simulink model "Efficiency_Map_SR_Validation_Sim"  (R2017b)
settings: Solver=VariableStepAuto  StartTime=0.0  StopTime=10.0  RelTol=1e-3
values from neighbouring files (symbols this model uses):
  ap00 = -69.58    [Efficiency_Map_Validation.m]    (also in Efficiency_Maps.m)
  ap01 = 11.22    [Efficiency_Map_Validation.m]    (also in Efficiency_Maps.m)
  ap02 = -0.1665    [Efficiency_Map_Validation.m]    (also in Efficiency_Maps.m)
  ap03 = 0.0006218    [Efficiency_Map_Validation.m]    (also in Efficiency_Maps.m)
  ap10 = 0.5123    [Efficiency_Map_Validation.m]    (also in Efficiency_Maps.m)
  ap11 = 0.009736    [Efficiency_Map_Validation.m]    (also in Efficiency_Maps.m)
  ap12 = 0.0003316    [Efficiency_Map_Validation.m]    (also in Efficiency_Maps.m)
  ap20 = -0.0007943    [Efficiency_Map_Validation.m]    (also in Efficiency_Maps.m)
  ap21 = -4.587e-07    [Efficiency_Map_Validation.m]    (also in Efficiency_Maps.m)
  ap30 = 3.794e-07    [Efficiency_Map_Validation.m]    (also in Efficiency_Maps.m)
  motor_speed = mtr_speed_rad(j)    [Efficiency_Map_Validation.m]
  motor_torque = mtr_torque(i)    [Efficiency_Map_Validation.m]
settings Model: Creator=Robert Wygant  LastModifiedBy=Robert Wygant

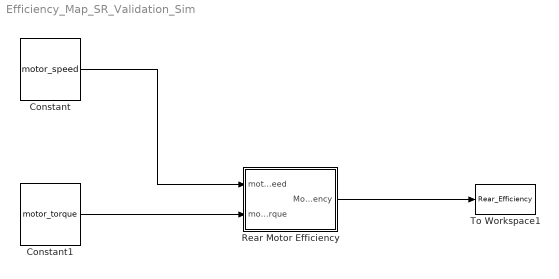
== system Efficiency_Map_SR_Validation_Sim ==
  Constant : Constant  Value=motor_speed
  Constant1 : Constant  Value=motor_torque
  Rear Motor Efficiency : Subsystem
      mask Display:
      | color('green')
      | disp("Motor Efficiency")
  To Workspace1 : ToWorkspace  VariableName=Rear_Efficiency  SampleTime=-1
      settings: MaxDataPoints=1  Save2DSignal=2-D array (concatenate along first dimension)
  wires:
  Constant/1 -> Rear Motor Efficiency/1(motor_speed)
  Constant1/1 -> Rear Motor Efficiency/2(motor_torque)
  Rear Motor Efficiency/1(Motor_efficiency) -> To Workspace1/1

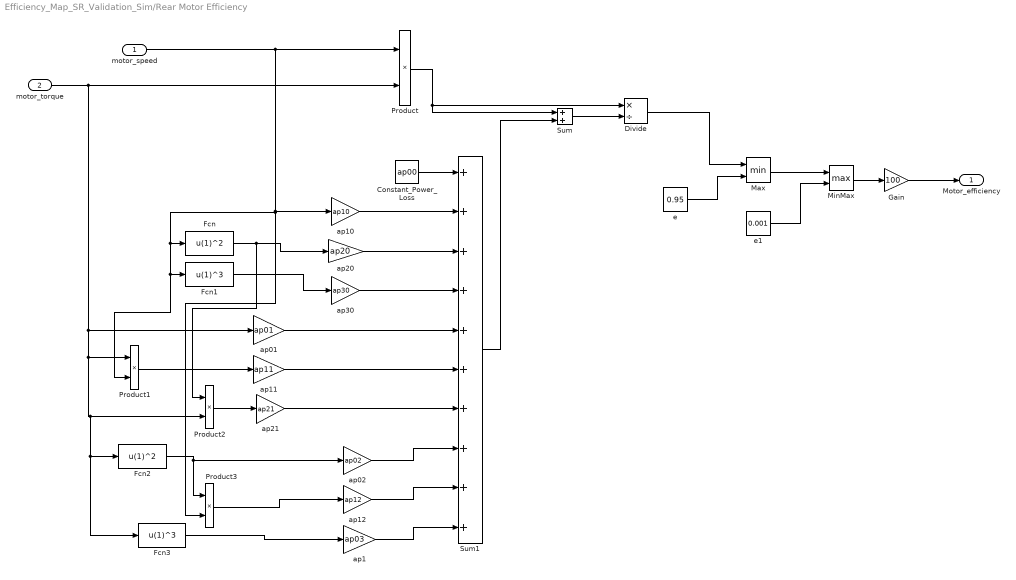
== system Efficiency_Map_SR_Validation_Sim/Rear Motor Efficiency ==
  motor_speed : Inport
  motor_torque : Inport  Port=2
  Constant_Power_Loss : Constant  Value=ap00
  Divide : Product  Inputs=*/
  Fcn : Fcn  Expr=u(1)^2
  Fcn1 : Fcn  Expr=u(1)^3
  Fcn2 : Fcn  Expr=u(1)^2
  Fcn3 : Fcn  Expr=u(1)^3
  Gain : Gain  Gain=100
  Max : MinMax  Inputs=2
  MinMax : MinMax  Function=max  Inputs=2
  Product{,1..3} (4 alike) : Product
  Sum : Sum
  Sum1 : Sum  Inputs=++++++++++
  ap01 : Gain  Gain=ap01
  ap02 : Gain  Gain=ap02
  ap1 : Gain  Gain=ap03
  ap10 : Gain  Gain=ap10
  ap11 : Gain  Gain=ap11
  ap12 : Gain  Gain=ap12
  ap20 : Gain  Gain=ap20
  ap21 : Gain  Gain=ap21
  ap30 : Gain  Gain=ap30
  e : Constant  Value=0.95
  e1 : Constant  Value=0.001
  Motor_efficiency : Outport
  wires:
  e/1 -> Max/2
  Fcn3/1 -> ap1/1
  ap1/1 -> Sum1/10
  ap12/1 -> Sum1/9
  Product3/1 -> ap12/1
  motor_torque/1 -> Product/2, Product1/1, Product2/2, Fcn2/1, Fcn3/1, ap01/1
  ap01/1 -> Sum1/5
  ap11/1 -> Sum1/6
  ap21/1 -> Sum1/7
  ap02/1 -> Sum1/8
  Fcn2/1 -> ap02/1, Product3/1
  Product2/1 -> ap21/1
  Product1/1 -> ap11/1
  ap30/1 -> Sum1/4
  Fcn1/1 -> ap30/1
  Fcn/1 -> ap20/1, Product2/1
  ap20/1 -> Sum1/3
  ap10/1 -> Sum1/2
  Constant_Power_Loss/1 -> Sum1/1
  motor_speed/1 -> Product/1, Product3/2, Fcn/1, Fcn1/1, Product1/2, ap10/1
  Divide/1 -> Max/1
  Sum1/1 -> Sum/2
  Sum/1 -> Divide/2
  Product/1 -> Divide/1, Sum/1
  Max/1 -> MinMax/1
  MinMax/1 -> Gain/1
  e1/1 -> MinMax/2
  Gain/1 -> Motor_efficiency/1
